simulink model "sample_load"  (Simulink 6.4)
settings: Solver=ode23s  StartTime=0.0  StopTime=10  RelTol=1e-3
libraries: dc_motor_lib x1
settings Model: Creator=raarenst  LastModifiedBy=raarenst

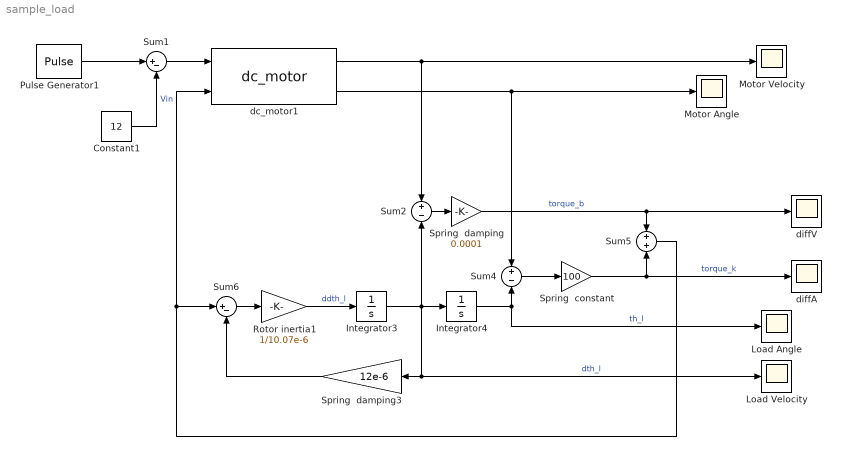
== system sample_load ==
  Constant1 : Constant  Value=12  OutDataType=sfix(16)  ConRadixGroup=Use specified scaling  OutScaling=2^0  SampleTime=inf  FramePeriod=inf
  Integrator3 : Integrator
  Integrator4 : Integrator
  Load Angle : Scope
      settings: SaveName=ScopeData2
  Load Velocity : Scope
  Motor Angle : Scope
  Motor Velocity : Scope
      settings: SaveName=ScopeData4
  Pulse Generator1 : DiscretePulseGenerator  PulseType=Time based  Amplitude=24  Period=10  PulseWidth=50
  Rotor inertia1 : Gain  Gain=1/10.07e-6
  Spring  constant : Gain  Gain=100
  Spring  damping : Gain  Gain=0.0001
  Spring  damping3 : Gain  Orientation=left  Gain=12e-6
  Sum1 : Sum  Inputs=|+-
  Sum2 : Sum  Inputs=+-
  Sum4 : Sum  Inputs=+-
  Sum5 : Sum
  Sum6 : Sum  Inputs=|+-
  dc_motor1 : dc_motor_lib/dc_motor  SystemSampleTime=-1  Rm=2.06  Lm=0.000238  Kb=1/((406*2*pi)/60)  Kt=0.0235  Jm=1.07e-6  bm=12e-7
  diffA : Scope
      settings: SaveName=ScopeData5
  diffV : Scope
      settings: SaveName=ScopeData3
  wires:
  Integrator3/1 -> Integrator4/1, Sum2/2, Spring  damping3/1, Load Velocity/1  "dth_l"
  Integrator4/1 -> Sum4/2, Load Angle/1  "th_l"
  Rotor inertia1/1 -> Integrator3/1  "ddth_l"
  Sum2/1 -> Spring  damping/1
  Sum4/1 -> Spring  constant/1
  Spring  damping/1 -> Sum5/1, diffV/1  "torque_b"
  Spring  constant/1 -> Sum5/2, diffA/1  "torque_k"
  Sum5/1 -> Sum6/1, dc_motor1/2
  Sum6/1 -> Rotor inertia1/1
  Spring  damping3/1 -> Sum6/2
  dc_motor1/1 -> Sum2/1, Motor Velocity/1
  dc_motor1/2 -> Sum4/1, Motor Angle/1
  Pulse Generator1/1 -> Sum1/1
  Constant1/1 -> Sum1/2  "Vin"
  Sum1/1 -> dc_motor1/1
